simulink model "stateflow4"  (R2015a)
settings: Solver=ode3  StartTime=0.0  StopTime=inf  RelTol=1e-3
libraries: legoev3lib x3
settings Model: SimulationMode=external  ExtModeTrigDuration=2  Creator=USER  LastModifiedBy=Keshav
settings OptimizationCC: OptimizeModelRefInitCode=on  LifeSpan=1
settings DebuggingCC: UnderspecifiedInitializationDetection=Classic  MergeDetectMultiDrivingBlocksExec=none
settings HardwareCC: ProdLargestAtomicInteger=Long  ProdLargestAtomicFloat=Float  ProdEndianess=LittleEndian  ProdHWDeviceType=ARM Compatible->ARM 9
settings RTWCC: SystemTargetFile=realtime.tlc  GenerateMakefile=off  TemplateMakefile=realtime.tmf  Description=Run on Target Hardware  RTWVerbose=off
settings ERTTargetCC: CombineOutputUpdateFcns=off  ExtMode=on  ExtModeMexArgs='192.168.0.105' 0 17725 30  ERTSrcFileBannerTemplate=realtime_code_template.cgt  ERTHdrFileBannerTemplate=realtime_code_template.cgt  ERTDataSrcFileTemplate=realtime_code_template.cgt  ERTDataHdrFileTemplate=realtime_code_template.cgt  ERTCustomFileTemplate=realtime_file_process.tlc

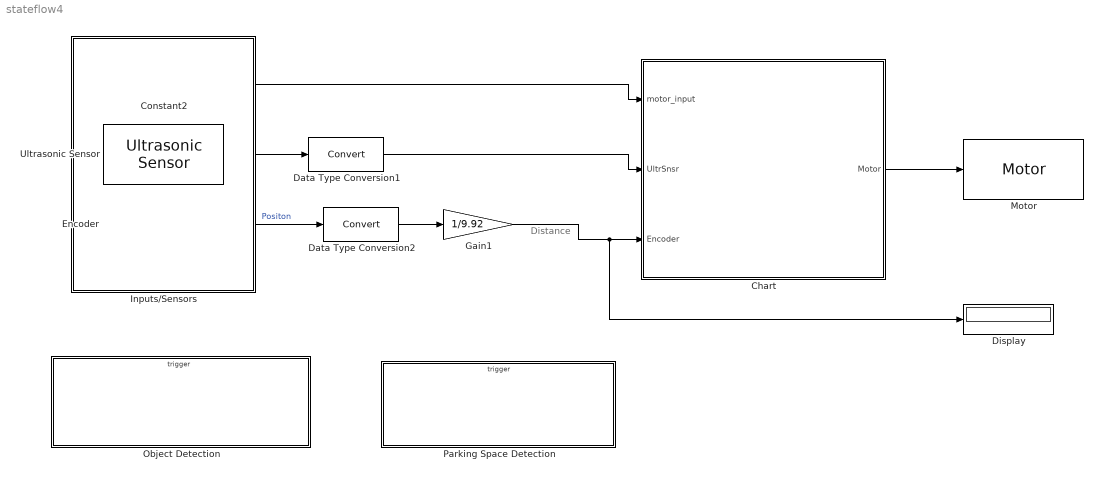
== system stateflow4 ==
  note: Distance
  Chart : Stateflow chart  TreatAsAtomicUnit=on
  Constant2 : Constant  Value=30
  Data Type Conversion1 : DataTypeConversion
  Data Type Conversion2 : DataTypeConversion
  Display : Display
  Encoder : legoev3lib/Encoder  portNumber=A  opMode=No reset  sampleTime=0.01
  Gain1 : Gain  Gain=1/9.92
  Inputs/Sensors : Subsystem
  Motor : legoev3lib/Motor  sportNumber=A  sstopAction=Brake
  Object Detection : Subsystem  TreatAsAtomicUnit=on
  Parking Space Detection : Subsystem  TreatAsAtomicUnit=on
  Ultrasonic Sensor : legoev3lib/Ultrasonic Sensor  PortNumber=1  sampleTime=0.01
  wires:
  Ultrasonic Sensor/1 -> Data Type Conversion1/1
  Data Type Conversion2/1 -> Gain1/1
  Data Type Conversion1/1 -> Chart/2(UltrSnsr)
  Constant2/1 -> Chart/1(motor_input)
  Chart/1(Motor) -> Motor/1
  Encoder/1 -> Data Type Conversion2/1  "Positon"
  Gain1/1 -> Display/1, Chart/3(Encoder)

== system stateflow4/Inputs//Sensors ==

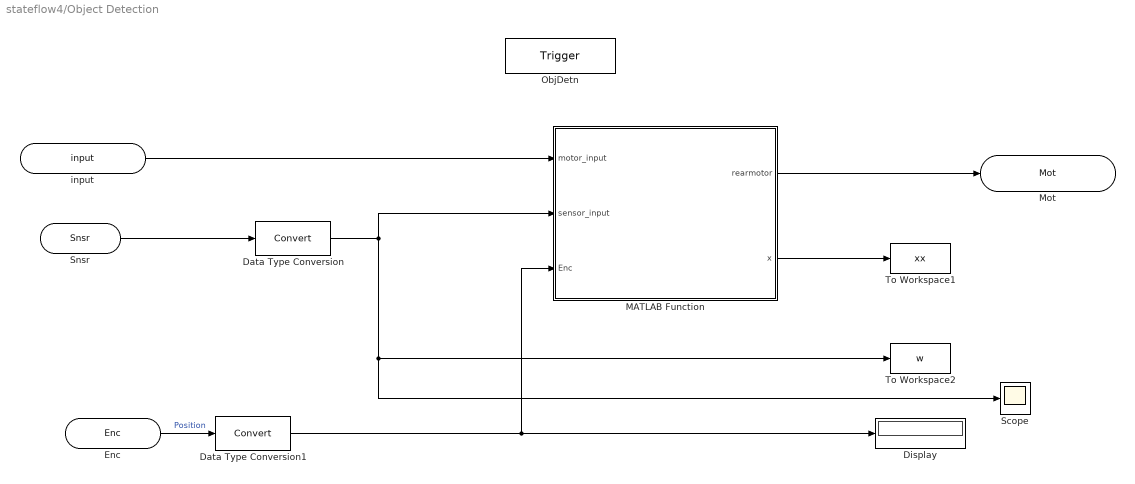
== system stateflow4/Object Detection ==
  ObjDetn : TriggerPort  TriggerType=function-call  IsSimulinkFunction=on  FunctionName=ObjDetn
  Data Type Conversion : DataTypeConversion
  Data Type Conversion1 : DataTypeConversion
  Display : Display
  MATLAB Function : MATLAB Function  TreatAsAtomicUnit=on
  Scope : Scope
      settings: YMin=2.85  YMax=3.15
  To Workspace1 : ToWorkspace  VariableName=xx  SampleTime=-1
  To Workspace2 : ToWorkspace  VariableName=w  SampleTime=-1
  input : ArgIn  DisableCoverage=on  ArgumentName=input
  Snsr : ArgIn  DisableCoverage=on  Port=2  ArgumentName=Snsr
  Enc : ArgIn  DisableCoverage=on  Port=3  ArgumentName=Enc
  Mot : ArgOut  DisableCoverage=on  ArgumentName=Mot
  wires:
  Data Type Conversion/1 -> To Workspace2/1, Scope/1, MATLAB Function/2(sensor_input)
  MATLAB Function/1(rearmotor) -> Mot/1
  Enc/1 -> Data Type Conversion1/1  "Position"
  Snsr/1 -> Data Type Conversion/1
  input/1 -> MATLAB Function/1(motor_input)
  Data Type Conversion1/1 -> Display/1, MATLAB Function/3(Enc)
  MATLAB Function/2(x) -> To Workspace1/1

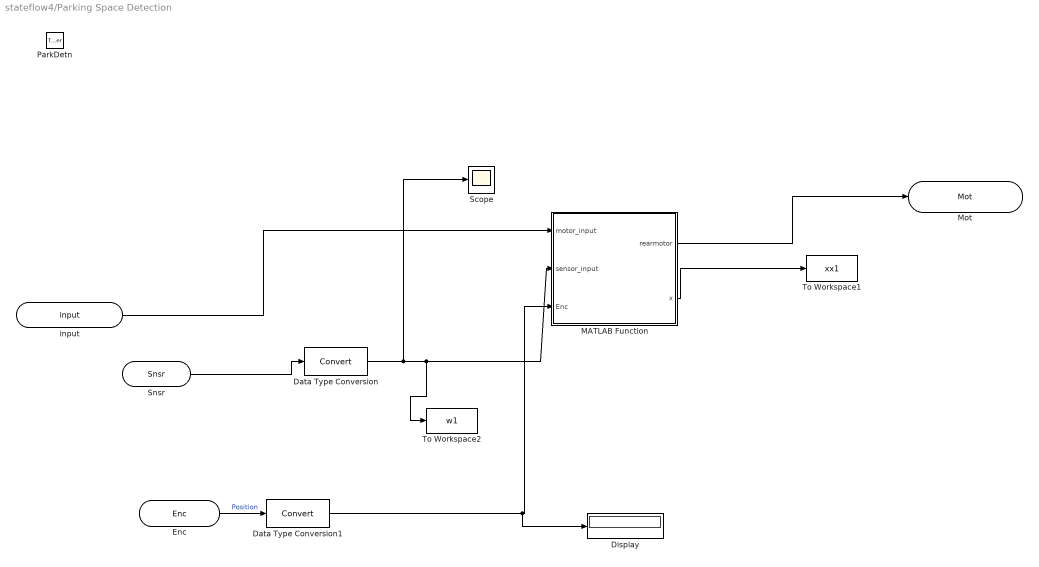
== system stateflow4/Parking Space Detection ==
  ParkDetn : TriggerPort  TriggerType=function-call  IsSimulinkFunction=on  FunctionName=ParkDetn
  Data Type Conversion : DataTypeConversion
  Data Type Conversion1 : DataTypeConversion
  Display : Display
  MATLAB Function : MATLAB Function  TreatAsAtomicUnit=on
  Scope : Scope
      settings: YMin=3  YMax=3
  To Workspace1 : ToWorkspace  VariableName=xx1  SampleTime=-1
  To Workspace2 : ToWorkspace  VariableName=w1  SampleTime=-1
  input : ArgIn  DisableCoverage=on  ArgumentName=input
  Snsr : ArgIn  DisableCoverage=on  Port=2  ArgumentName=Snsr
  Enc : ArgIn  DisableCoverage=on  Port=3  ArgumentName=Enc
  Mot : ArgOut  DisableCoverage=on  ArgumentName=Mot
  wires:
  Data Type Conversion/1 -> Scope/1, To Workspace2/1, MATLAB Function/2(sensor_input)
  MATLAB Function/1(rearmotor) -> Mot/1
  Enc/1 -> Data Type Conversion1/1  "Position"
  Snsr/1 -> Data Type Conversion/1
  input/1 -> MATLAB Function/1(motor_input)
  Data Type Conversion1/1 -> Display/1, MATLAB Function/3(Enc)
  MATLAB Function/2(x) -> To Workspace1/1

== matlab function stateflow4/Parking Space Detection/MATLAB Function ==
  data: motor_input input; sensor_input input; rearmotor output; x output; Enc input
function [rearmotor,x]= fcn(motor_input,sensor_input,Enc)
%#codegen
%d = z
%u = 0; %Encoder reset
x = Enc;
length2=0;
%reset11=0;
%state3=0;
if(sensor_input>24)&&(sensor_input<=60)
    rearmotor=motor_input-20;
    if (Enc>=73)&&(Enc<=74)
        length2=Enc;
        rearmotor=0;
%        reset11=1;
    %    state3=1;        
    end
    %elseif(sensor_input>20)&&(sensor_input<=35)
 %   rearmotor=motor_input;
%else(sensor_input>24)&&(sensor_input<=61)
 %   x = u;
  %  rearmotor=motor_input-10;
   % u=1;    
    %if(sensor_input<=20)
    %    rearmotor=0;   
%else((sensor_input-z)>2)||((sensor_input-z)<-2)
   % rearmotor=0;
else
    rearmotor=motor_input-10;

%state3=0;
end



end

== matlab function stateflow4/Object Detection/MATLAB Function ==
  data: motor_input input; sensor_input input; rearmotor output; x output; Enc input
function [rearmotor,x]= fcn(motor_input,sensor_input,Enc)
%#codegen
%d = z
%u = 0; %Encoder reset
x = Enc;
lenght2=0;
%reset1=0;
%state2=0;
if(sensor_input>4)&&(sensor_input<=20)
    rearmotor=motor_input;
    if (Enc>=30)&&(Enc<=31)
        length1=30;
        rearmotor=0;
%        reset1=1;
     %   state2=1;        
    end
    %elseif(sensor_input>20)&&(sensor_input<=35)
 %   rearmotor=motor_input;
%else(sensor_input>24)&&(sensor_input<=61)
 %   x = u;
  %  rearmotor=motor_input-10;
   % u=1;    
    %if(sensor_input<=20)
    %    rearmotor=0;   
%else((sensor_input-z)>2)||((sensor_input-z)<-2)
   % rearmotor=0;
else
    rearmotor=0;
    %state2=0;
end



end

== stateflow chart stateflow4/Chart ==
  (default) -> (junction 47) : {Motor = ObjDetn(motor_input,UltrSnsr,Encoder)}
  (junction 47) -> (junction 48) : [Encoder>=30 && UltrSnsr>24]
      | {Motor = ParkDetn(motor_input,UltrSnsr,Encoder)}
  data: motor_input input; Motor output; UltrSnsr input; Encoder input
